simulink model "euler_equation_dave"  (R2021b)
settings: Solver=VariableStepAuto  StartTime=0.0  StopTime=30  MaxStep=0.01  RelTol=1e-3
values from neighbouring files (symbols this model uses):
  a = 2.4501e+4    (= 24501)    [heliocentric_plot.m]    (also in parameters_euler_equations_dave.m = 10500)
  e = 0.6665    [heliocentric_plot.m]    (also in parameters_euler_equations_dave.m = 0)
  Euler0131 = [0 pi/4 0]'    [parameters_euler_equations_dave.m]
  Euler0312 = [pi/4, 0, 0]'    [parameters_euler_equations_dave.m]
  h_versor = h ./ (h_norm)    [parameters_euler_equations_dave.m]
  I = [I_x_body, I_y_body, I_z_body]    [parameters_euler_equations_dave.m]
  i_0 = 0    [parameters_euler_equations_dave.m]
  J = diag (I)    [parameters_euler_equations_dave.m]
  J_inv = inv(J)    [parameters_euler_equations_dave.m]
  Mat_g = g .* S * 1e-09    [ghnorm.m]
  Mat_gsv = gsv .* S*  1e-09    [ghnorm.m]
  Mat_h = h .* S * 1e-09    [ghnorm.m]
  Mat_hsv = hsv .* S*  1e-09    [ghnorm.m]
  muP = astroConstants(13)    [parameters_euler_equations_dave.m]
  n = mat(:, 1)    [ghnorm.m]    (also in parameters_euler_equations_dave.m = 2*pi/T)
  N = max(mat (:, 2))    [ghnorm.m]    (also in parameters_euler_equations_dave.m = [n1 n2 n3 n4 n5 n6])
  n_sun = 2*pi/(365*24*3600)    (= 1.99238499086e-07)    [parameters_euler_equations_dave.m]    (also in srp.m = 1.99102127766e-07)
  R_sun = 149600000    [parameters_euler_equations_dave.m]
  Sat_dim = [a_body b_body c_body]    [parameters_euler_equations_dave.m]
  star1_in = [Sx(1); Sy(1); Sz(1)]    [parameters_euler_equations_dave.m]    (also in stars.m)
  star2_in = [Sx(2); Sy(2); Sz(2)]    [parameters_euler_equations_dave.m]    (also in stars.m)
  star3_in = [Sx(3); Sy(3); Sz(3)]    [parameters_euler_equations_dave.m]    (also in stars.m)
  theta_g0 = 0    [parameters_euler_equations_dave.m]
  true_anomaly0 = 0    [parameters_euler_equations_dave.m]
  Ts = 0.1    [parameters_euler_equations_dave.m]
  w0 = [wx, wy, wz]    [parameters_euler_equations_dave.m]
undefined symbols (not defined in the file or in its folder): A_SB, g_mat, h_mat, init_mjd2000, magnetic_torque, r0, t0, v0, vec_norm, we
libraries: sharedutil x13, vrlib x8, simulink_extras x6, sharedtransform x5, matrix_library x3, aerolibconvert2 x2, euler x1
(part 1 of 2)
settings Model: Creator=gargi  LastModifiedBy=white

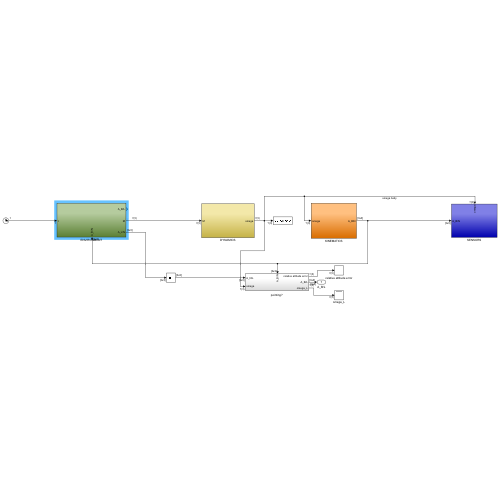
[thumbnail: Simulink's stored preview of the top-level diagram]
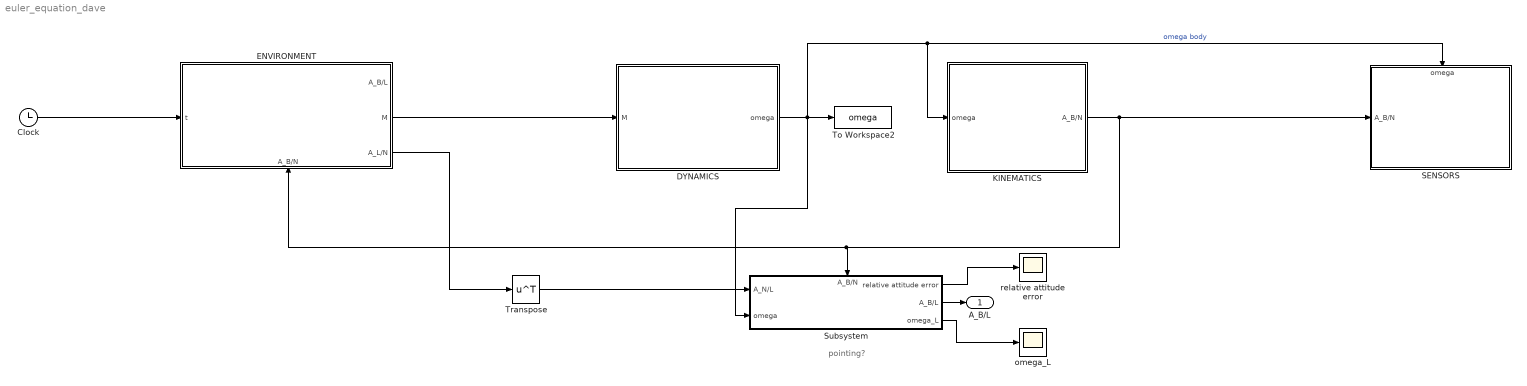
== system euler_equation_dave ==
  note: pointing?
  Clock : Clock
  DYNAMICS : Subsystem
  ENVIRONMENT : Subsystem
      settings: PortSchema="{\"entries\":[{\"content\":{\"sides\":[{\"content\":{\"connectorIds\":[\"In1\"]},\"type\":\"ConnectorPlacement.EquallySpacedRectSide\",\"uuid\":\"d64a220b-768f-41cc-b7f2-e1eda455b8cd\"},{\"content\":{\"connectorIds\":[\"Out1\",\"Out2\",\"Out3\"],\"side\":\"RIGHT\"},\"type\":\"ConnectorPlacement.EquallySpacedRectSide\",\"uuid\":\"0ef46d02-94aa-48e3-a1de-52aeb1814179\"},{\"content\":{\"connectorIds\":[],\"side\":\"TOP\"},\"type\":\"ConnectorPlacement.EquallySpacedRectSide\",\"uuid\":\"5be20339-a1cd-4229-b259-1b87d0a40b31\"},{\"content\":{\"connectorIds\":[\"In2\"],\"side\":\"BOTTOM\"},\"type\":\"ConnectorPlacement.EquallySpacedRectSide\",\"uuid\":\"00a59743-0b85-4da4-8c91-089e7d557d39\"}]},\"type\":\"ConnectorPlacement.EquallySpacedConnector\",\"uuid\":\"86e5647d-ad23-4d7e-bb48-80a2b4048e86\"}],\"packageUris\":[\"http://schema.mathworks.com/mf0/Connector/R2020b\"],\"version\":\"1.0\"}"
  KINEMATICS : Subsystem
  SENSORS : Subsystem
      settings: PortSchema="{\"entries\":[{\"content\":{\"sides\":[{\"content\":{\"connectorIds\":[\"In1\"]},\"type\":\"ConnectorPlacement.EquallySpacedRectSide\",\"uuid\":\"6630fbbb-ea2b-425d-8575-1523cccd696b\"},{\"content\":{\"connectorIds\":[],\"side\":\"RIGHT\"},\"type\":\"ConnectorPlacement.EquallySpacedRectSide\",\"uuid\":\"07965b78-7ff0-471d-b26c-4fdda1f5d939\"},{\"content\":{\"connectorIds\":[\"In2\"],\"side\":\"TOP\"},\"type\":\"ConnectorPlacement.EquallySpacedRectSide\",\"uuid\":\"40925145-5336-49f5-bea5-25b26df713fa\"}]},\"type\":\"ConnectorPlacement.EquallySpacedConnector\",\"uuid\":\"3c2f6bfd-4663-43ab-9562-77b2e75e3828\"}],\"packageUris\":[\"http://schema.mathworks.com/mf0/Connector/R2020b\"],\"version\":\"1.0\"}"
  Subsystem : Subsystem
      settings: PortSchema="{\"entries\":[{\"content\":{\"sides\":[{\"content\":{\"connectorIds\":[\"In1\",\"In2\"]},\"type\":\"ConnectorPlacement.EquallySpacedRectSide\",\"uuid\":\"153df774-f390-4caa-8633-d509b8614b34\"},{\"content\":{\"connectorIds\":[\"Out1\",\"Out2\",\"Out3\"],\"side\":\"RIGHT\"},\"type\":\"ConnectorPlacement.EquallySpacedRectSide\",\"uuid\":\"2b0b455d-aa9a-478c-9b12-a1c7f0c2757e\"},{\"content\":{\"connectorIds\":[\"In3\"],\"side\":\"TOP\"},\"type\":\"ConnectorPlacement.EquallySpacedRectSide\",\"uuid\":\"e181ccf7-3891-483c-b413-5a84ce39d941\"}]},\"type\":\"ConnectorPlacement.EquallySpacedConnector\",\"uuid\":\"4911c07f-3db9-4f8f-9913-f96600dbf3f5\"}],\"packageUris\":[\"http://schema.mathworks.com/mf0/Connector/R2020b\"],\"version\":\"1.0\"}"
  To Workspace2 : ToWorkspace  VariableName=omega  SampleTime=-1
  Transpose : Math  Operator=transpose  SaturateOnIntegerOverflow=on
  omega_L : Scope
  relative attitude error : Scope
  A_B/L : Outport
  wires:
  DYNAMICS/1(omega) -> To Workspace2/1, SENSORS/2(omega), KINEMATICS/1(omega), Subsystem/2(omega)  "omega body"
  KINEMATICS/1(A_B/N) -> SENSORS/1(A_B/N), Subsystem/3(A_B/N), ENVIRONMENT/2(A_B/N)
  Transpose/1 -> Subsystem/1(A_N/L)
  Subsystem/1(relative attitude error) -> relative attitude error/1
  Subsystem/2(A_B/L) -> A_B/L/1
  Subsystem/3(omega_L) -> omega_L/1
  ENVIRONMENT/3(A_L/N) -> Transpose/1
  ENVIRONMENT/2(M) -> DYNAMICS/1(M)
  Clock/1 -> ENVIRONMENT/1(t)

== system euler_equation_dave/DYNAMICS ==
  M : Inport
  Cross Product : matrix_library/Cross Product
      settings: SourceProductBaseCode=SL
  Integrator : Integrator  InitialCondition=w0
  J : Gain  Gain=J  Multiplication=Matrix(K*u)
  J inv : Gain  Gain=J_inv  Multiplication=Matrix(K*u)
  Sum : Sum  Inputs=|++
  omega : Outport
  wires:
  Integrator/1 -> J/1, Cross Product/2, omega/1
  J/1 -> Cross Product/1
  J inv/1 -> Integrator/1  "omega_dot"
  Cross Product/1 -> Sum/1  "J w cross w"
  Sum/1 -> J inv/1
  M/1 -> Sum/2

== system euler_equation_dave/ENVIRONMENT ==
  note: A is from INERTIAL to LVLH
  t : Inport
  A_B/N : Inport  Port=2
  ECEF : Subsystem
  GRADIENT TORQUE : Subsystem
  MAGNETIC TORQUE : Subsystem
  "ORBITAL MECHANICS " : Subsystem
  SRP : Subsystem  Commented=on
  SUN : Subsystem
  Scope : Scope
  Scope1 : Scope
  Sum : Sum  Inputs=+++
  To create A_L/N : Subsystem
  h : Constant  Value=h_versor
  "to create c1, c2, c3" : Subsystem
  A_B/L : Outport
  M : Outport  Port=2
  A_L/N : Outport  Port=3
  wires:
  "to create c1, c2, c3"/1("c1, c2, c3") -> GRADIENT TORQUE/1("c1, c2, c3")  "c1,c2,c3"
  A_B/N/1 -> SRP/1(A_BN), SUN/1(A_BN), MAGNETIC TORQUE/2(A_B/N), "to create c1, c2, c3"/1(A_B/N)
  "to create c1, c2, c3"/2(A_B/L) -> A_B/L/1
  GRADIENT TORQUE/1(M_GG) -> Sum/1
  Sum/1 -> M/1
  To create A_L/N/1(A_L/N) -> Scope/1, A_L/N/1, "to create c1, c2, c3"/2(A_L/N)
  h/1 -> To create A_L/N/1(h_versor)
  "ORBITAL MECHANICS "/2(R) -> GRADIENT TORQUE/2(R)  "in km"
  "ORBITAL MECHANICS "/1(r_N_versor) -> To create A_L/N/2(r_N_versor)
  t/1 -> SUN/2(t), MAGNETIC TORQUE/3(t), SRP/2(t)
  SRP/1(Output) -> Scope1/1, Sum/3
  "ORBITAL MECHANICS "/4(r_N) -> MAGNETIC TORQUE/1(r_N)  "r_N in km"
  MAGNETIC TORQUE/1(M_Magn) -> Sum/2

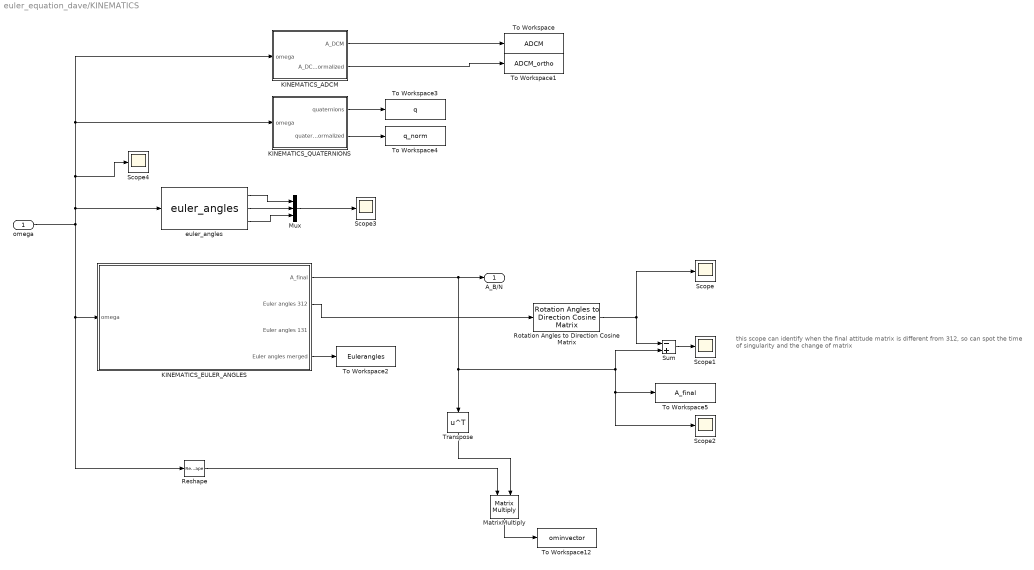
== system euler_equation_dave/KINEMATICS ==
  note: this scope can identify when the final attitude
      | matrix is different from 312, so can spot
      | the time of singularity and the change of matrix
  omega : Inport
  KINEMATICS_ADCM : Subsystem
  KINEMATICS_EULER_ANGLES : Subsystem
  KINEMATICS_QUATERNIONS : Subsystem
  MatrixMultiply : Product  Multiplication=Matrix(*)
  Mux : Mux  Inputs=3
  Reshape : Reshape  OutputDimensionality=Row vector (2-D)
  Rotation Angles to Direction Cosine Matrix : sharedtransform/Rotation Angles to Direction Cosine Matrix  rotationOrder=ZXY  aMode=aMode
      settings: SourceProductBaseCode=AE,PW,DR,MT,UV,VE
  Scope{,1..4} (5 alike) : Scope
  Sum : Sum  Inputs=-+
  To Workspace : ToWorkspace  VariableName=ADCM  SampleTime=-1
  To Workspace1 : ToWorkspace  VariableName=ADCM_ortho  SampleTime=-1
  To Workspace12 : ToWorkspace  VariableName=ominvector  SampleTime=-1
  To Workspace2 : ToWorkspace  VariableName=Eulerangles  SampleTime=-1
  To Workspace3 : ToWorkspace  VariableName=q  SampleTime=-1
  To Workspace4 : ToWorkspace  VariableName=q_norm  SampleTime=-1
  To Workspace5 : ToWorkspace  VariableName=A_final  SampleTime=-1
  Transpose : Math  Operator=transpose  SaturateOnIntegerOverflow=on
  euler_angles : euler/euler_angles  SystemSampleTime=-1  VariantActivationTime=update diagram  Latency=0  AutoFrameSizeCalculation=off
      link override phi_block/Integrator: InitialCondition=pi/4
      link override psi_block/Integrator: InitialCondition=0
      link override theta_block/Integrator: InitialCondition=0
  A_B/N : Outport
  wires:
  Transpose/1 -> MatrixMultiply/2
  Reshape/1 -> MatrixMultiply/1
  KINEMATICS_QUATERNIONS/2(quaternions normalized) -> To Workspace4/1
  omega/1 -> euler_angles/1, Scope4/1, KINEMATICS_ADCM/1(omega), KINEMATICS_QUATERNIONS/1(omega), KINEMATICS_EULER_ANGLES/1(omega), Reshape/1
  MatrixMultiply/1 -> To Workspace12/1
  KINEMATICS_ADCM/2(A_DCM orthonormalized) -> To Workspace1/1
  KINEMATICS_QUATERNIONS/1(quaternions) -> To Workspace3/1
  KINEMATICS_EULER_ANGLES/1(A_final) -> Scope2/1, To Workspace5/1, Sum/2, Transpose/1, A_B/N/1
  KINEMATICS_ADCM/1(A_DCM) -> To Workspace/1
  Sum/1 -> Scope1/1
  KINEMATICS_EULER_ANGLES/2(Euler angles 312) -> Rotation Angles to Direction Cosine Matrix/1
  Rotation Angles to Direction Cosine Matrix/1 -> Scope/1, Sum/1
  KINEMATICS_EULER_ANGLES/4(Euler angles merged) -> To Workspace2/1
  euler_angles/1 -> Mux/1
  euler_angles/2 -> Mux/2
  euler_angles/3 -> Mux/3
  Mux/1 -> Scope3/1

== system euler_equation_dave/SENSORS ==
  A_B/N : Inport
  omega : Inport  Port=2
  ATTITUDE DETERMINATION FOR GYROSCOPES : Subsystem  Commented=on
  ATTITUDE DETERMINATION FOR STAR SENSOR : Subsystem  Commented=on
  GYROSCOPES : Subsystem  Commented=on
  STAR SENSOR : Subsystem  Commented=on
  wires:
  omega/1 -> GYROSCOPES/1(omega)
  A_B/N/1 -> STAR SENSOR/1(A_B/N)
  GYROSCOPES/1(omega measured) -> ATTITUDE DETERMINATION FOR GYROSCOPES/1(omega measured)
  ATTITUDE DETERMINATION FOR GYROSCOPES/1(Attitude final measured) -> ?
  ATTITUDE DETERMINATION FOR GYROSCOPES/2(Euler angles merged measured) -> ?
  STAR SENSOR/1(star1_meas) -> ?
  STAR SENSOR/2(star2_meas) -> ?

== system euler_equation_dave/Subsystem ==
  A_N/L : Inport
  omega : Inport  Port=2
  A_B/N : Inport  Port=3
  MatrixMultiply : Product  Multiplication=Matrix(*)
  MatrixMultiply1 : Product  Multiplication=Matrix(*)
  MatrixMultiply2 : Product  Multiplication=Matrix(*)
  Scope : Scope
  Sum : Sum  Inputs=+-
  Transpose1 : Math  Operator=transpose  SaturateOnIntegerOverflow=on
  relative attitude error : Outport
  A_B/L : Outport  Port=2
  omega_L : Outport  Port=3
  wires:
  MatrixMultiply/1 -> Transpose1/1, MatrixMultiply2/1, A_B/L/1  "A_B/L"
  Transpose1/1 -> MatrixMultiply1/1  "A_L/B"
  omega/1 -> Sum/1, MatrixMultiply1/2  "omega"
  MatrixMultiply1/1 -> omega_L/1, MatrixMultiply2/2, Sum/2  "omega_L"
  A_B/N/1 -> MatrixMultiply/1
  A_N/L/1 -> MatrixMultiply/2
  Sum/1 -> relative attitude error/1

== system euler_equation_dave/ENVIRONMENT/ECEF ==
  In1 : Inport
  Out1 : Outport
  wires:
  In1/1 -> Out1/1

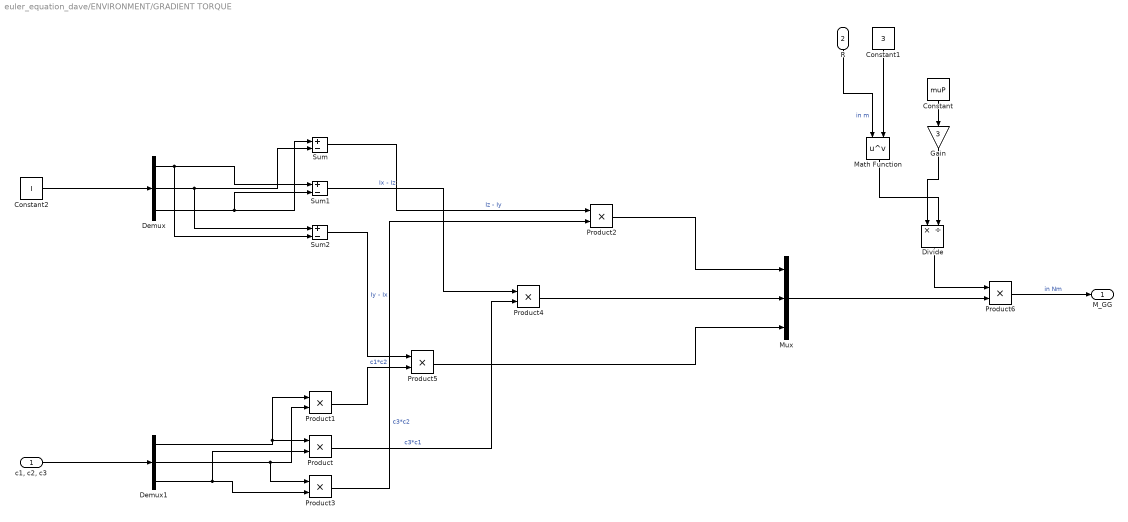
== system euler_equation_dave/ENVIRONMENT/GRADIENT TORQUE ==
  "c1, c2, c3" : Inport
  R : Inport  Port=2
  Constant : Constant  Value=muP
  Constant1 : Constant  Value=3
  Constant2 : Constant  Value=I
  Demux : Demux  Outputs=3
  Demux1 : Demux  Outputs=3
  Divide : Product  Inputs=*/
  Gain : Gain  Gain=3
  Math Function : Math  Operator=pow  SaturateOnIntegerOverflow=on
  Mux : Mux  Inputs=3
  Product{,1..6} (7 alike) : Product
  Sum : Sum  Inputs=+-
  Sum1 : Sum  Inputs=+-
  Sum2 : Sum  Inputs=+-
  M_GG : Outport
  wires:
  Constant/1 -> Gain/1
  Gain/1 -> Divide/1
  R/1 -> Math Function/1  "in m"
  Constant1/1 -> Math Function/2
  Math Function/1 -> Divide/2
  Constant2/1 -> Demux/1
  Demux/1 -> Sum2/2, Sum1/1
  Demux/2 -> Sum2/1, Sum/2
  Demux/3 -> Sum/1, Sum1/2
  Demux1/1 -> Product1/1, Product/1
  Demux1/2 -> Product1/2, Product3/1
  Demux1/3 -> Product/2, Product3/2
  "c1, c2, c3"/1 -> Demux1/1
  Sum/1 -> Product2/1  "Iz - Iy"
  Sum1/1 -> Product4/1  "Ix - Iz"
  Product3/1 -> Product2/2  "c3*c2"
  Product/1 -> Product4/2  "c3*c1"
  Product1/1 -> Product5/2  "c1*c2"
  Sum2/1 -> Product5/1  "Iy - Ix"
  Product2/1 -> Mux/1
  Product5/1 -> Mux/3
  Product4/1 -> Mux/2
  Divide/1 -> Product6/1
  Mux/1 -> Product6/2
  Product6/1 -> M_GG/1  "in Nm"

== system euler_equation_dave/ENVIRONMENT/MAGNETIC TORQUE ==
  r_N : Inport
  A_B/N : Inport  Port=2
  t : Inport  Port=3
  Subsystem : Subsystem  Commented=on
  magnetic_torque : Subsystem  AncestorBlock=magnetic_torque/magnetic_torque
  M_Magn : Outport
  wires:
  r_N/1 -> magnetic_torque/1(r_N)
  A_B/N/1 -> magnetic_torque/2(A_N_to_B)
  magnetic_torque/1(magnetic_torque) -> M_Magn/1
  t/1 -> magnetic_torque/3(t)

== system euler_equation_dave/ENVIRONMENT/ORBITAL MECHANICS  ==
  Scope1 : Scope
  Sum : Sum  Inputs=+-
  cartesian position integrator : Subsystem
  "cartesian position with keplerian formulas " : Subsystem
  r_N_versor : Outport
  R : Outport  Port=2
  cartesian position : Outport  Port=3
  r_N : Outport  Port=4
  wires:
  Sum/1 -> Scope1/1
  cartesian position integrator/1(carteasion_position_versor) -> Sum/2
  cartesian position integrator/2(cartesian position) -> cartesian position/1
  "cartesian position with keplerian formulas "/3(r_N_versor) -> Sum/1, r_N_versor/1
  "cartesian position with keplerian formulas "/1(R) -> R/1
  "cartesian position with keplerian formulas "/2(rN) -> r_N/1

== system euler_equation_dave/ENVIRONMENT/SRP ==
  A_BN : Inport
  t : Inport  Port=2
  MATLAB Function : MATLAB Function  TreatAsAtomicUnit=on
  N_surfaces : Constant  Value=N
  Reshape : Reshape
  Sat_dim : Constant  Value=Sat_dim
  Output : Outport
  wires:
  Sat_dim/1 -> MATLAB Function/1(Sat_dim)
  t/1 -> MATLAB Function/4(t)  "clock"
  A_BN/1 -> MATLAB Function/3(A_BN)
  N_surfaces/1 -> MATLAB Function/2(N)
  MATLAB Function/1(M) -> Reshape/1
  Reshape/1 -> Output/1

== system euler_equation_dave/ENVIRONMENT/SUN ==
  A_BN : Inport
  t : Inport  Port=2
  Constant2 : Constant  Value=eps
  Cos : Trigonometry  Operator=cos
  Cos1 : Trigonometry  Operator=cos
  Gain : Gain  Gain=R_sun
  MatrixMultiply : Product  Multiplication=Matrix(*)
  Mux : Mux  Inputs=3
  Normalize Vector : vrlib/Utilities/Normalize Vector  maxzero=0
  Product1 : Product
  Product2 : Product
  Sin : Trigonometry
  Sin1 : Trigonometry
  "n_sun " : Gain  Gain=n_sun
  S_N : Outport  VectorParamsAs1DForOutWhenUnconnected=off
  S_B : Outport  Port=2
  wires:
  Mux/1 -> Gain/1
  Product2/1 -> Mux/3
  Product1/1 -> Mux/2
  Cos/1 -> Mux/1
  t/1 -> "n_sun "/1
  Constant2/1 -> Sin1/1, Cos1/1
  Sin1/1 -> Product2/2
  Sin/1 -> Product1/1, Product2/1
  "n_sun "/1 -> Sin/1, Cos/1
  Cos1/1 -> Product1/2
  Gain/1 -> Normalize Vector/1
  A_BN/1 -> MatrixMultiply/1
  Normalize Vector/1 -> MatrixMultiply/2, S_N/1
  MatrixMultiply/1 -> S_B/1

== system euler_equation_dave/ENVIRONMENT/To create A_L//N ==
  h_versor : Inport
  r_N_versor : Inport  Port=2
  Create 3x3 Matrix : sharedutil/Create 3x3 Matrix  aMode=aMode
      settings: SourceProductBaseCode=AE,PW,DR,MT,UV,VE
  Demux : Demux  Outputs=3
  Demux1 : Demux  Outputs=3
  Demux2 : Demux  Outputs=3
  Scope : Scope
  To comput theta_versor : Subsystem
  A_L/N : Outport
  wires:
  Demux2/3 -> Create 3x3 Matrix/9
  Demux/1 -> Create 3x3 Matrix/1
  r_N_versor/1 -> To comput theta_versor/2(r_N_versor), Demux/1
  Demux/3 -> Create 3x3 Matrix/3
  To comput theta_versor/1(theta_versor) -> Demux1/1
  Demux2/2 -> Create 3x3 Matrix/8
  Demux1/1 -> Create 3x3 Matrix/4
  Demux2/1 -> Create 3x3 Matrix/7
  Demux/2 -> Create 3x3 Matrix/2
  Demux1/2 -> Create 3x3 Matrix/5
  Demux1/3 -> Create 3x3 Matrix/6
  h_versor/1 -> Demux2/1, To comput theta_versor/1(h_versor)
  Create 3x3 Matrix/1 -> Scope/1, A_L/N/1

== system euler_equation_dave/ENVIRONMENT/to create c1, c2, c3 ==
  note: from LVLH to Body frame
  A_B/N : Inport
  A_L/N : Inport  Port=2
  Constant : Constant  Value=[1 0 0]'
  MatrixMultiply : Product  Multiplication=Matrix(*)
  MatrixMultiply1 : Product  Multiplication=Matrix(*)
  Transpose : Math  Operator=transpose  SaturateOnIntegerOverflow=on
  "c1, c2, c3" : Outport
  A_B/L : Outport  Port=2
  wires:
  MatrixMultiply/1 -> A_B/L/1, MatrixMultiply1/1
  A_L/N/1 -> Transpose/1
  Constant/1 -> MatrixMultiply1/2
  Transpose/1 -> MatrixMultiply/2
  MatrixMultiply1/1 -> "c1, c2, c3"/1  "c1, c2, c3"
  A_B/N/1 -> MatrixMultiply/1

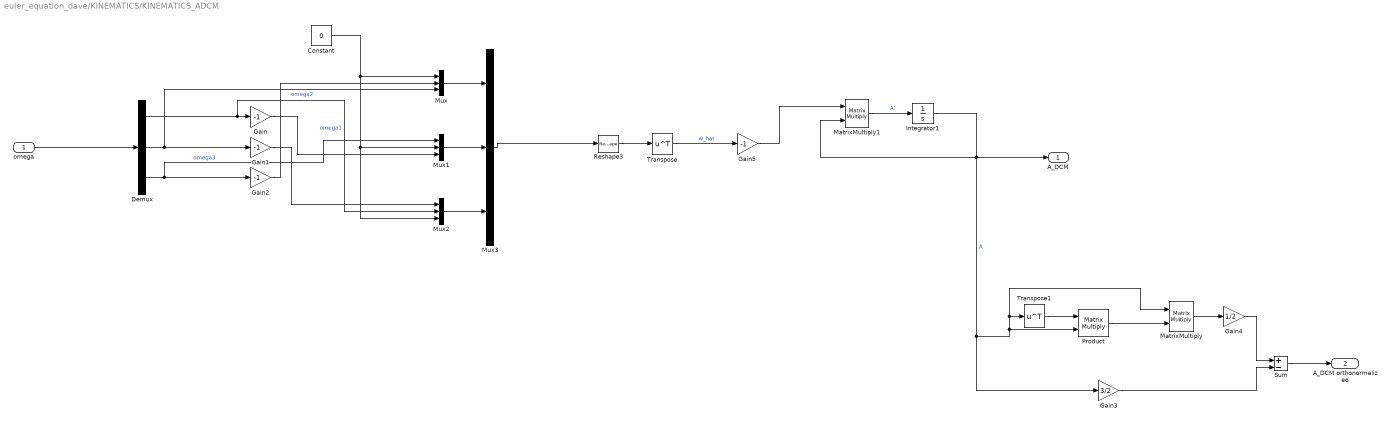
== system euler_equation_dave/KINEMATICS/KINEMATICS_ADCM ==
  omega : Inport
  Constant : Constant  Value=0
  Demux : Demux  Outputs=3
  Gain{,1..2,5} (4 alike) : Gain  Gain=-1
  Gain3 : Gain  Gain=3/2
  Gain4 : Gain  Gain=1/2
  Integrator1 : Integrator  InitialCondition=eye(3)
  MatrixMultiply : Product  Multiplication=Matrix(*)
  MatrixMultiply1 : Product  Multiplication=Matrix(*)
  Mux{,1..3} (4 alike) : Mux  Inputs=3
  Product : Product  Multiplication=Matrix(*)
  Reshape3 : Reshape  OutputDimensionality=Customize  OutputDimensions=[3 3]
  Sum : Sum  Inputs=+-
  Transpose : Math  Operator=transpose  SaturateOnIntegerOverflow=on
  Transpose1 : Math  Operator=transpose  SaturateOnIntegerOverflow=on
  A_DCM : Outport
  A_DCM orthonormalized : Outport  Port=2
  wires:
  Mux/1 -> Mux3/1
  Demux/1 -> Gain/1, Mux2/2  "omega1"
  Constant/1 -> Mux2/3, Mux1/2, Mux/1
  Gain/1 -> Mux1/3
  Mux3/1 -> Reshape3/1
  Gain1/1 -> Mux2/1
  Demux/2 -> Mux/3, Gain1/1  "omega2"
  Mux1/1 -> Mux3/2
  Demux/3 -> Mux1/1, Gain2/1  "omega3"
  Mux2/1 -> Mux3/3
  Gain2/1 -> Mux/2
  Reshape3/1 -> Transpose/1
  omega/1 -> Demux/1
  Transpose/1 -> Gain5/1  "w_hat"
  Integrator1/1 -> MatrixMultiply1/2, A_DCM/1, MatrixMultiply/1, Transpose1/1, Product/2, Gain3/1  "A"
  Transpose1/1 -> Product/1
  Gain4/1 -> Sum/1
  Gain3/1 -> Sum/2
  Sum/1 -> A_DCM orthonormalized/1
  MatrixMultiply/1 -> Gain4/1
  Product/1 -> MatrixMultiply/2
  Gain5/1 -> MatrixMultiply1/1
  MatrixMultiply1/1 -> Integrator1/1  "A'"

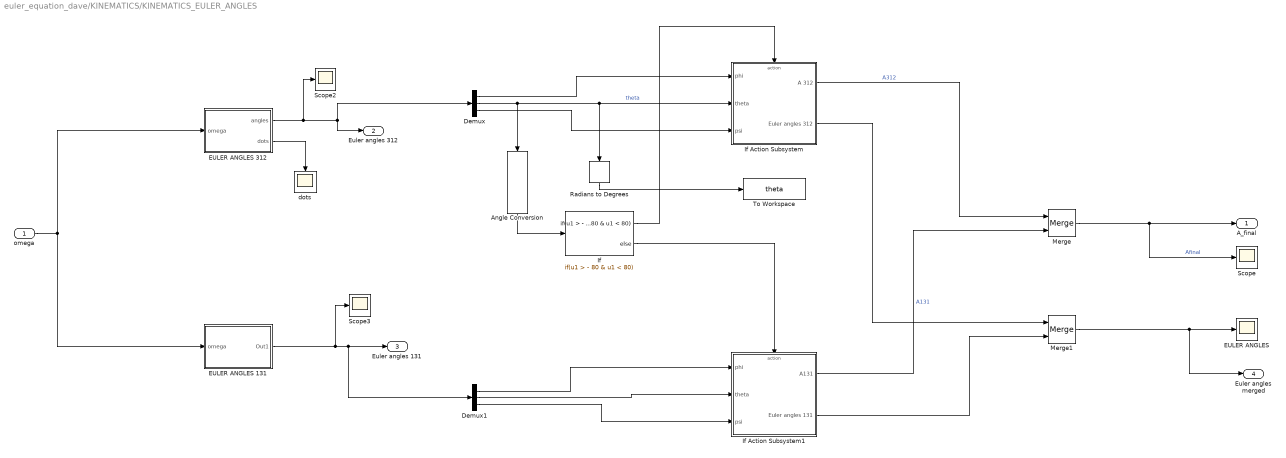
== system euler_equation_dave/KINEMATICS/KINEMATICS_EULER_ANGLES ==
  omega : Inport
  Angle Conversion : aerolibconvert2/Angle Conversion  IU=rad  OU=deg
  Demux : Demux  Outputs=3
  Demux1 : Demux  Outputs=3
  EULER ANGLES : Scope
  EULER ANGLES 131 : Subsystem
  EULER ANGLES 312 : Subsystem
  If : If  IfExpression=u1 > - 80 & u1 < 80
  If Action Subsystem : Subsystem  TreatAsAtomicUnit=on
  If Action Subsystem1 : Subsystem  TreatAsAtomicUnit=on
  Merge : Merge
  Merge1 : Merge
  Radians to Degrees : simulink_extras/Transformations/Radians to Degrees
  Scope : Scope
  Scope2 : Scope
  Scope3 : Scope
  To Workspace : ToWorkspace  VariableName=theta  SaveFormat=Timeseries  SampleTime=-1
  dots : Scope
  A_final : Outport
  Euler angles 312 : Outport  Port=2
  Euler angles 131 : Outport  Port=3
  Euler angles merged : Outport  Port=4
  wires:
  Angle Conversion/1 -> If/1
  If/2 -> If Action Subsystem1/Action
  If/1 -> If Action Subsystem/Action
  If Action Subsystem1/1(A131) -> Merge/2  "A131"
  If Action Subsystem/1(A 312) -> Merge/1  "A312"
  Merge/1 -> Scope/1, A_final/1  "Afinal"
  omega/1 -> EULER ANGLES 312/1(omega), EULER ANGLES 131/1(omega)
  Demux/2 -> Radians to Degrees/1, If Action Subsystem/2(theta), Angle Conversion/1  "theta"
  Demux/1 -> If Action Subsystem/1(phi)
  Demux/3 -> If Action Subsystem/3(psi)
  EULER ANGLES 312/1(angles) -> Scope2/1, Euler angles 312/1, Demux/1
  Demux1/1 -> If Action Subsystem1/1(phi)
  Demux1/2 -> If Action Subsystem1/2(theta)
  Demux1/3 -> If Action Subsystem1/3(psi)
  EULER ANGLES 131/1(Out1) -> Scope3/1, Euler angles 131/1, Demux1/1
  If Action Subsystem/2(Euler angles 312) -> Merge1/1
  If Action Subsystem1/2(Euler angles 131) -> Merge1/2
  Merge1/1 -> Euler angles merged/1, EULER ANGLES/1
  EULER ANGLES 312/2(dots) -> dots/1
  Radians to Degrees/1 -> To Workspace/1

== system euler_equation_dave/KINEMATICS/KINEMATICS_QUATERNIONS ==
  omega : Inport
  Demux : Demux  Outputs=3
  Gain : Gain  Gain=1/2
  Integrator : Integrator  InitialCondition=[0 0 0 1]
  Normalize Vector : vrlib/Utilities/Normalize Vector  maxzero=0
  Product : Product
  Product1 : Product
  Product2 : Product
  Product3 : Product  Multiplication=Matrix(*)
  Sum : Sum  Inputs=+++
  mat1 : Constant  Value=[0 0 0 1; 0 0 1 0; 0 -1 0 0; -1 0 0 0]
  mat2 : Constant  Value=[0 0 -1 0; 0 0 0 1; 1 0 0 0; 0 -1 0 0]
  mat3 : Constant  Value=[0 1 0 0; -1 0 0 0; 0 0 0 1; 0 0 -1 0]
  quaternions : Outport
  quaternions normalized : Outport  Port=2
  wires:
  mat1/1 -> Product/1
  Demux/1 -> Product/2
  Product/1 -> Sum/1
  mat2/1 -> Product1/1
  Demux/2 -> Product1/2
  Product1/1 -> Sum/2
  Demux/3 -> Product2/2
  mat3/1 -> Product2/1
  Product2/1 -> Sum/3
  Sum/1 -> Gain/1  "OMEGA"
  omega/1 -> Demux/1
  Gain/1 -> Product3/1
  Product3/1 -> Integrator/1  "q'"
  Integrator/1 -> quaternions/1, Normalize Vector/1  "q"
  Normalize Vector/1 -> Product3/2, quaternions normalized/1

== system euler_equation_dave/SENSORS/ATTITUDE DETERMINATION FOR GYROSCOPES ==
  note: star sensor
  omega measured : Inport
  Angle Conversion : aerolibconvert2/Angle Conversion  IU=rad  OU=deg
  Demux : Demux  Outputs=3
  Demux1 : Demux  Outputs=3
  EULER ANGLES : Scope
  EULER ANGLES 131 : Subsystem
  EULER ANGLES 312 : Subsystem
  If : If  IfExpression=u1 > - 80 & u1 < 80
  If Action Subsystem : Subsystem  TreatAsAtomicUnit=on
  If Action Subsystem1 : Subsystem  TreatAsAtomicUnit=on
  Merge : Merge
  Merge1 : Merge
  Scope : Scope
  Scope2 : Scope
  Scope3 : Scope
  dots : Scope
  Attitude final measured : Outport
  Euler angles merged measured : Outport  Port=2
  wires:
  If Action Subsystem1/1(A131) -> Merge/2  "A131"
  EULER ANGLES 312/2(dots) -> dots/1
  EULER ANGLES 131/1(Out1) -> Scope3/1, Demux1/1
  Demux1/2 -> If Action Subsystem1/2(theta)
  Demux1/3 -> If Action Subsystem1/3(psi)
  Demux/1 -> If Action Subsystem/1(phi)
  Demux/3 -> If Action Subsystem/3(psi)
  Merge/1 -> Scope/1, Attitude final measured/1  "Afinal"
  If Action Subsystem1/2(Euler angles 131) -> Merge1/2
  Demux1/1 -> If Action Subsystem1/1(phi)
  omega measured/1 -> EULER ANGLES 312/1(omega), EULER ANGLES 131/1(omega)
  Merge1/1 -> Euler angles merged measured/1, EULER ANGLES/1
  If Action Subsystem/2(Euler angles 312) -> Merge1/1
  Demux/2 -> If Action Subsystem/2(theta), Angle Conversion/1  "theta"
  If Action Subsystem/1(A 312) -> Merge/1  "A312"
  EULER ANGLES 312/1(angles) -> Scope2/1, Demux/1
  Angle Conversion/1 -> If/1
  If/1 -> If Action Subsystem/Action
  If/2 -> If Action Subsystem1/Action

== system euler_equation_dave/SENSORS/ATTITUDE DETERMINATION FOR STAR SENSOR ==
  In1 : Inport
  Out1 : Outport
  wires:
  In1/1 -> Out1/1

== system euler_equation_dave/SENSORS/GYROSCOPES ==
  omega : Inport
  Bias : Constant  Value=[1; 1; 1]*0.0035
  Degrees to Radians : simulink_extras/Transformations/Degrees to Radians
  Gain : Gain  Gain=1/3600
  Product : Product
  Random Number : RandomNumber  Mean=[0 0 0 ]'  Variance=[1 1 1]'  Seed=[0 0 0]'  SampleTime=0.1
  Scope1 : Scope
  Scope2 : Scope
  Sigma_n : Subsystem
  Sum : Sum  Inputs=+++
  Sum1 : Sum  Inputs=+-
  omega measured : Outport
  wires:
  Bias/1 -> Degrees to Radians/1  "b in deg/h"
  Degrees to Radians/1 -> Gain/1
  Sum/1 -> omega measured/1, Sum1/1
  omega/1 -> Scope2/1, Sum1/2, Sum/2
  Gain/1 -> Sum/3
  Sum1/1 -> Scope1/1
  Random Number/1 -> Product/2
  Product/1 -> Sum/1
  Sigma_n/1(Out1) -> Product/1

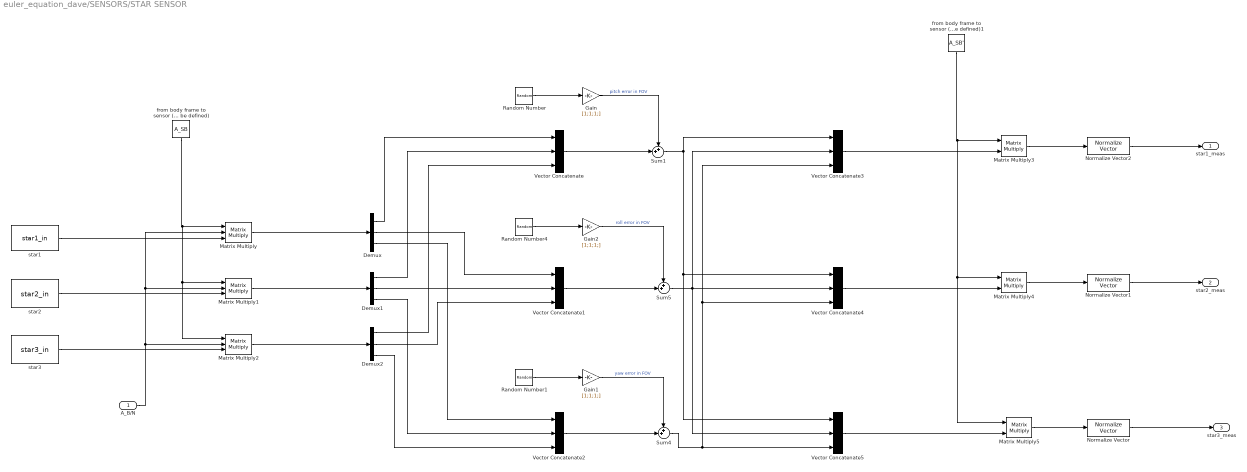
== system euler_equation_dave/SENSORS/STAR SENSOR ==
  A_B/N : Inport
  Demux : Demux  Outputs=3
  Demux1 : Demux  Outputs=3
  Demux2 : Demux  Outputs=3
  Gain : Gain  Gain=[1;1;1;]
  Gain1 : Gain  Gain=[1;1;1;]
  Gain2 : Gain  Gain=[1;1;1;]
  Matrix Multiply : Product  Inputs=3  Multiplication=Matrix(*)
  Matrix Multiply1 : Product  Inputs=3  Multiplication=Matrix(*)
  Matrix Multiply2 : Product  Inputs=3  Multiplication=Matrix(*)
  Matrix Multiply3 : Product  Multiplication=Matrix(*)
  Matrix Multiply4 : Product  Multiplication=Matrix(*)
  Matrix Multiply5 : Product  Multiplication=Matrix(*)
  Normalize Vector : vrlib/Utilities/Normalize Vector  maxzero=0
  Normalize Vector1 : vrlib/Utilities/Normalize Vector  maxzero=0
  Normalize Vector2 : vrlib/Utilities/Normalize Vector  maxzero=0
  Random Number : RandomNumber  Variance=((8.25/3600)*(pi/180))^2  SampleTime=0.1
  Random Number1 : RandomNumber  Variance=((8.25/3600)*(pi/180))^2  SampleTime=0.1
  Random Number4 : RandomNumber  Variance=((11.1/3600)*(pi/180))^2  SampleTime=0.1
  Sum1 : Sum  Inputs=++|
  Sum4 : Sum  Inputs=++|
  Sum5 : Sum  Inputs=++|
  Vector Concatenate{,1..5} (6 alike) : Concatenate  NumInputs=3
  from body frame to sensor (yet to be defined) : Constant  Value=A_SB
  from body frame to sensor (yet to be defined)1 : Constant  Value=A_SB'
  star1 : Constant  Value=star1_in
  star2 : Constant  Value=star2_in
  star3 : Constant  Value=star3_in
  star1_meas : Outport
  star2_meas : Outport  Port=2
  star3_meas : Outport  Port=3
  wires:
  Demux/1 -> Vector Concatenate/1
  Demux1/1 -> Vector Concatenate/2
  Demux2/1 -> Vector Concatenate/3
  Demux/2 -> Vector Concatenate1/1
  Demux1/2 -> Vector Concatenate1/2
  Demux2/2 -> Vector Concatenate1/3
  Demux/3 -> Vector Concatenate2/1
  Demux1/3 -> Vector Concatenate2/2
  Demux2/3 -> Vector Concatenate2/3
  Matrix Multiply/1 -> Demux/1
  Matrix Multiply1/1 -> Demux1/1
  Matrix Multiply2/1 -> Demux2/1
  A_B/N/1 -> Matrix Multiply/2, Matrix Multiply1/2, Matrix Multiply2/2
  from body frame to sensor (yet to be defined)/1 -> Matrix Multiply2/1, Matrix Multiply1/1, Matrix Multiply/1
  star1/1 -> Matrix Multiply/3
  star2/1 -> Matrix Multiply1/3
  star3/1 -> Matrix Multiply2/3
  Vector Concatenate/1 -> Sum1/2
  Random Number/1 -> Gain/1
  Gain/1 -> Sum1/1  "pitch error in FOV"
  Random Number4/1 -> Gain2/1
  Gain2/1 -> Sum5/1  "roll error in FOV"
  Vector Concatenate1/1 -> Sum5/2
  Random Number1/1 -> Gain1/1
  Gain1/1 -> Sum4/1  "yaw error in FOV"
  Vector Concatenate2/1 -> Sum4/2
  Sum1/1 -> Vector Concatenate3/1, Vector Concatenate5/1, Vector Concatenate4/1
  Sum5/1 -> Vector Concatenate5/2, Vector Concatenate4/2, Vector Concatenate3/2
  Sum4/1 -> Vector Concatenate4/3, Vector Concatenate3/3, Vector Concatenate5/3
  Vector Concatenate3/1 -> Matrix Multiply3/2
  Vector Concatenate4/1 -> Matrix Multiply4/2
  Vector Concatenate5/1 -> Matrix Multiply5/2
  from body frame to sensor (yet to be defined)1/1 -> Matrix Multiply3/1, Matrix Multiply4/1, Matrix Multiply5/1
  Matrix Multiply3/1 -> Normalize Vector2/1
  Normalize Vector2/1 -> star1_meas/1
  Matrix Multiply4/1 -> Normalize Vector1/1
  Normalize Vector1/1 -> star2_meas/1
  Matrix Multiply5/1 -> Normalize Vector/1
  Normalize Vector/1 -> star3_meas/1

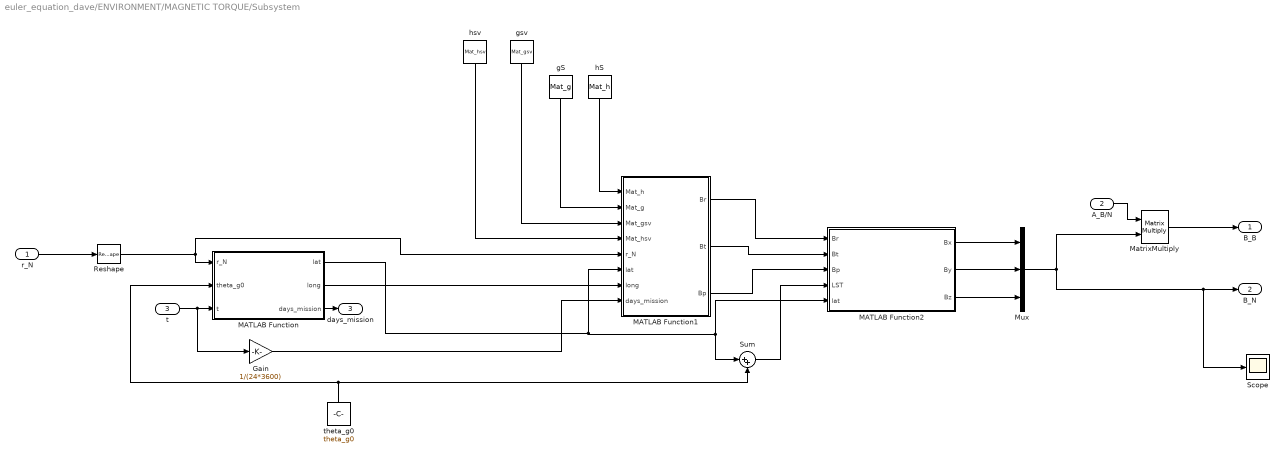
== system euler_equation_dave/ENVIRONMENT/MAGNETIC TORQUE/Subsystem ==
  r_N : Inport
  A_B/N : Inport  Port=2
  t : Inport  Port=3
  Gain : Gain  Gain=1/(24*3600)
  MATLAB Function : MATLAB Function  TreatAsAtomicUnit=on
  MATLAB Function1 : MATLAB Function  TreatAsAtomicUnit=on
  MATLAB Function2 : MATLAB Function  TreatAsAtomicUnit=on
  MatrixMultiply : Product  Multiplication=Matrix(*)
  Mux : Mux  Inputs=3
  Reshape : Reshape  OutputDimensionality=Row vector (2-D)
  Scope : Scope
  Sum : Sum  Inputs=|++
  gS : Constant  Value=Mat_g
  gsv : Constant  Value=Mat_gsv
  hS : Constant  Value=Mat_h
  hsv : Constant  Value=Mat_hsv
  theta_g0 : Constant  Value=theta_g0
  B_B : Outport
  B_N : Outport  Port=2
  days_mission : Outport  Port=3
  wires:
  MATLAB Function/2(long) -> MATLAB Function1/7(long)
  A_B/N/1 -> MatrixMultiply/1
  MATLAB Function2/1(Bx) -> Mux/1
  MATLAB Function2/2(By) -> Mux/2
  MATLAB Function2/3(Bz) -> Mux/3
  MATLAB Function1/1(Br) -> MATLAB Function2/1(Br)
  theta_g0/1 -> MATLAB Function/2(theta_g0), Sum/2
  MATLAB Function1/2(Bt) -> MATLAB Function2/2(Bt)
  MATLAB Function1/3(Bp) -> MATLAB Function2/3(Bp)
  MATLAB Function/1(lat) -> MATLAB Function1/6(lat), Sum/1, MATLAB Function2/5(lat)
  Sum/1 -> MATLAB Function2/4(LST)
  MatrixMultiply/1 -> B_B/1
  gsv/1 -> MATLAB Function1/3(Mat_gsv)
  t/1 -> Gain/1, MATLAB Function/3(t)
  MATLAB Function/3(days_mission) -> days_mission/1
  Mux/1 -> MatrixMultiply/2, B_N/1, Scope/1
  Reshape/1 -> MATLAB Function1/5(r_N), MATLAB Function/1(r_N)
  gS/1 -> MATLAB Function1/2(Mat_g)
  hS/1 -> MATLAB Function1/1(Mat_h)
  Gain/1 -> MATLAB Function1/8(days_mission)
  hsv/1 -> MATLAB Function1/4(Mat_hsv)
  r_N/1 -> Reshape/1

== system euler_equation_dave/ENVIRONMENT/MAGNETIC TORQUE/magnetic_torque ==
  note: degrees
  note: degrees
  note: M = m x B
  note: degrees
  r_N : Inport
  A_N_to_B : Inport  Port=2
  t : Inport  Port=3
  MATLAB Function : MATLAB Function  TreatAsAtomicUnit=on
  N_to_B : Product  Multiplication=Matrix(*)
  constants : Subsystem
  gaussian_coefficients : Subsystem
  m : Constant  Value=[0.01; 0.05; 0.01]
  mjd2000_block : Subsystem
  nT_to_T : Gain  Gain=1e-9
  r_N_to_lat_lon_lst : Subsystem
  theta_g : Subsystem
  to_torque : matrix_library/Cross Product
      settings: SourceProductBaseCode=SL
  magnetic_torque : Outport
  wires:
  nT_to_T/1 -> N_to_B/2  "B_N"
  gaussian_coefficients/2(h_mat) -> MATLAB Function/7(h_mat)
  mjd2000_block/1(mjd2000) -> MATLAB Function/5(mjd2000)
  gaussian_coefficients/1(g_mat) -> MATLAB Function/6(g_mat)
  constants/1(we) -> theta_g/2(we)  "we"
  constants/2(t0) -> theta_g/3(t0)  "t0"
  constants/3(theta_g0) -> theta_g/4(theta_g0)  "theta_g0"
  theta_g/1(theta_g) -> r_N_to_lat_lon_lst/2(theta_g)  "theta_g"
  r_N_to_lat_lon_lst/4(alpha) -> MATLAB Function/4(alpha)  "alpha"
  r_N_to_lat_lon_lst/1(r) -> MATLAB Function/1(r)  "r"
  m/1 -> to_torque/1  "m"
  to_torque/1 -> magnetic_torque/1  "magnetic_torque"
  N_to_B/1 -> to_torque/2  "B_B"
  MATLAB Function/1(B) -> nT_to_T/1  "B_N"
  A_N_to_B/1 -> N_to_B/1  "A_N_to_B"
  r_N_to_lat_lon_lst/3(lon) -> MATLAB Function/3(lon)  "lon"
  r_N_to_lat_lon_lst/2(lat) -> MATLAB Function/2(lat)  "lat"
  r_N/1 -> r_N_to_lat_lon_lst/1(r_N)  "r_N"
  t/1 -> theta_g/1(t)

== system euler_equation_dave/ENVIRONMENT/ORBITAL MECHANICS /cartesian position integrator ==
  Divide : Product  Inputs=*/
  Dot Product1 : DotProduct  InputSameDT=on  OutDataTypeStr=Inherit: Inherit via internal rule
  Gan : Gain  Gain=-muP
  Integrator : Integrator  InitialCondition=v0
  Integrator1 : Integrator  InitialCondition=r0
  Normalize Vector1 : vrlib/Utilities/Normalize Vector  maxzero=0
  carteasion_position_versor : Outport
  cartesian position : Outport  Port=2
  wires:
  Integrator1/1 -> cartesian position/1, Dot Product1/1, Dot Product1/2, Normalize Vector1/1  "cartesian position"
  Normalize Vector1/1 -> carteasion_position_versor/1, Divide/1  "r_versor"
  Divide/1 -> Gan/1
  Dot Product1/1 -> Divide/2  "r^2"
  Integrator/1 -> Integrator1/1
  Gan/1 -> Integrator/1  "acc"

== system euler_equation_dave/ENVIRONMENT/ORBITAL MECHANICS /cartesian position with keplerian formulas  ==
  Cos : Trigonometry  Operator=cos
  Cos1 : Trigonometry  Operator=cos
  Mux : Mux  Inputs=3
  Normalize Vector : vrlib/Utilities/Normalize Vector  maxzero=0
  Product : Product
  Product1 : Product
  Product2 : Product
  Scope : Scope
  Sin : Trigonometry
  Sin1 : Trigonometry
  eccentricity : Constant  Value=e
  inclination : Constant  Value=i_0
  to compute R : Subsystem
  to compute true anomaly : Subsystem
  R : Outport
  rN : Outport  Port=2
  r_N_versor : Outport  Port=3
  wires:
  inclination/1 -> Sin1/1, Cos1/1
  to compute true anomaly/1(theta) -> Sin/1, Cos/1, to compute R/2(theta)
  Sin/1 -> Product2/1, Product1/1
  to compute R/1(R) -> Scope/1, R/1, Product/1
  eccentricity/1 -> to compute R/1(e), to compute true anomaly/1(e)
  Cos/1 -> Mux/1
  Product/1 -> rN/1, Normalize Vector/1  "rN"
  Mux/1 -> Product/2
  Sin1/1 -> Product2/2
  Product1/1 -> Mux/2
  Cos1/1 -> Product1/2
  Product2/1 -> Mux/3
  Normalize Vector/1 -> r_N_versor/1

== system euler_equation_dave/ENVIRONMENT/To create A_L//N/To comput theta_versor ==
  h_versor : Inport
  r_N_versor : Inport  Port=2
  Cross Product : matrix_library/Cross Product
      settings: SourceProductBaseCode=SL
  Normalize Vector : vrlib/Utilities/Normalize Vector  maxzero=0
  theta_versor : Outport
  wires:
  Normalize Vector/1 -> Cross Product/2
  h_versor/1 -> Cross Product/1
  Cross Product/1 -> theta_versor/1
  r_N_versor/1 -> Normalize Vector/1

== system euler_equation_dave/KINEMATICS/KINEMATICS_EULER_ANGLES/EULER ANGLES 131 ==
  omega : Inport
  Integrator1 : Integrator  InitialCondition=Euler0131  WrapState=on
  Mux3 : Mux  Inputs=3
  PHI_DOT1 : Subsystem
  PSI DOT1 : Subsystem
  THETA DOT1 : Subsystem
  Out1 : Outport
  wires:
  Mux3/1 -> Integrator1/1
  PHI_DOT1/1(phi_dot) -> Mux3/2
  Integrator1/1 -> Out1/1, PSI DOT1/1(Euler angles), PHI_DOT1/1(euler angles), THETA DOT1/1(euler angles)
  THETA DOT1/1(theta_dot) -> Mux3/1
  omega/1 -> THETA DOT1/2(omega), PHI_DOT1/2(omega), PSI DOT1/2(omega)
  PSI DOT1/1(psi_dot) -> Mux3/3

== system euler_equation_dave/KINEMATICS/KINEMATICS_EULER_ANGLES/EULER ANGLES 312 ==
  omega : Inport
  Integrator : Integrator  InitialCondition=Euler0312  WrapState=on
  Mux2 : Mux  Inputs=3
  PHI_DOT : Subsystem
  PSI DOT : Subsystem
  THETA DOT : Subsystem
  angles : Outport
  dots : Outport  Port=2
  wires:
  omega/1 -> PSI DOT/2(omega), PHI_DOT/2(omega), THETA DOT/2(omega)
  Integrator/1 -> angles/1, PSI DOT/1(Euler angles), THETA DOT/1(euler angles), PHI_DOT/1(euler angles)
  PSI DOT/1(psi_dot) -> Mux2/3
  Mux2/1 -> dots/1, Integrator/1
  PHI_DOT/1(phi_dot) -> Mux2/1
  THETA DOT/1(theta_dot) -> Mux2/2

== system euler_equation_dave/KINEMATICS/KINEMATICS_EULER_ANGLES/If Action Subsystem ==
  phi : Inport
  theta : Inport  Port=2
  psi : Inport  Port=3
  Action Port : ActionPort  ActionPortLabel=if(u1 > - 80 & u1 < 80)
  A_312 : Subsystem
  Mux : Mux  Inputs=3
  Rotation Angles to Direction Cosine Matrix : sharedtransform/Rotation Angles to Direction Cosine Matrix  rotationOrder=ZXY  aMode=aMode
      settings: SourceProductBaseCode=AE,PW,DR,MT,UV,VE
  Scope : Scope
  Scope1 : Scope
  Sum : Sum  Inputs=-+
  A 312 : Outport
  Euler angles 312 : Outport  Port=2
  wires:
  A_312/1(A_312) -> Sum/2, A 312/1
  phi/1 -> Mux/1, A_312/1(phi)
  theta/1 -> Mux/2, A_312/2(theta)
  psi/1 -> Mux/3, A_312/3(psi)
  Mux/1 -> Rotation Angles to Direction Cosine Matrix/1, Euler angles 312/1
  Rotation Angles to Direction Cosine Matrix/1 -> Scope/1, Sum/1
  Sum/1 -> Scope1/1  "sottr"

== system euler_equation_dave/KINEMATICS/KINEMATICS_EULER_ANGLES/If Action Subsystem1 ==
  phi : Inport
  theta : Inport  Port=2
  psi : Inport  Port=3
  Action Port : ActionPort  ActionPortLabel=else
  A_131 : Subsystem
  Mux : Mux  Inputs=3
  Rotation Angles to Direction Cosine Matrix : sharedtransform/Rotation Angles to Direction Cosine Matrix  rotationOrder=XZX  aMode=aMode
      settings: SourceProductBaseCode=AE,PW,DR,MT,UV,VE
  Scope : Scope
  Sum : Sum  Inputs=+-
  A131 : Outport
  Euler angles 131 : Outport  Port=2
  wires:
  psi/1 -> Mux/3, A_131/3(psi)
  theta/1 -> Mux/2, A_131/2(theta)
  phi/1 -> Mux/1, A_131/1(phi)
  Mux/1 -> Rotation Angles to Direction Cosine Matrix/1, Euler angles 131/1
  Rotation Angles to Direction Cosine Matrix/1 -> Sum/1
  Sum/1 -> Scope/1  "sottr131"
  A_131/1(A_131) -> A131/1, Sum/2

== system euler_equation_dave/SENSORS/ATTITUDE DETERMINATION FOR GYROSCOPES/EULER ANGLES 131 ==
  omega : Inport
  Integrator1 : Integrator  InitialCondition=Euler0131  WrapState=on
  Mux3 : Mux  Inputs=3
  PHI_DOT1 : Subsystem
  PSI DOT1 : Subsystem
  THETA DOT1 : Subsystem
  Out1 : Outport
  wires:
  Mux3/1 -> Integrator1/1
  PHI_DOT1/1(phi_dot) -> Mux3/1
  Integrator1/1 -> Out1/1, PSI DOT1/1(Euler angles), THETA DOT1/1(euler angles), PHI_DOT1/1(euler angles)
  THETA DOT1/1(theta_dot) -> Mux3/2
  omega/1 -> PHI_DOT1/2(omega), THETA DOT1/2(omega), PSI DOT1/2(omega)
  PSI DOT1/1(psi_dot) -> Mux3/3

== system euler_equation_dave/SENSORS/ATTITUDE DETERMINATION FOR GYROSCOPES/EULER ANGLES 312 ==
  omega : Inport
  Integrator : Integrator  InitialCondition=Euler0312  WrapState=on
  Mux2 : Mux  Inputs=3
  PHI_DOT : Subsystem
  PSI DOT : Subsystem
  THETA DOT : Subsystem
  angles : Outport
  dots : Outport  Port=2
  wires:
  omega/1 -> PSI DOT/2(omega), PHI_DOT/2(omega), THETA DOT/2(omega)
  Integrator/1 -> angles/1, PSI DOT/1(Euler angles), THETA DOT/1(euler angles), PHI_DOT/1(euler angles)
  THETA DOT/1(theta_dot) -> Mux2/2
  PSI DOT/1(psi_dot) -> Mux2/3
  Mux2/1 -> dots/1, Integrator/1
  PHI_DOT/1(phi_dot) -> Mux2/1

== system euler_equation_dave/SENSORS/ATTITUDE DETERMINATION FOR GYROSCOPES/If Action Subsystem ==
  phi : Inport
  theta : Inport  Port=2
  psi : Inport  Port=3
  Action Port : ActionPort  ActionPortLabel=if(u1 > - 80 & u1 < 80)
  A_312 : Subsystem
  Mux : Mux  Inputs=3
  Rotation Angles to Direction Cosine Matrix : sharedtransform/Rotation Angles to Direction Cosine Matrix  rotationOrder=ZXY  aMode=aMode
      settings: SourceProductBaseCode=AE,PW,DR,MT,UV,VE
  Scope : Scope
  Scope1 : Scope
  Sum : Sum  Inputs=-+
  A 312 : Outport
  Euler angles 312 : Outport  Port=2
  wires:
  A_312/1(A_312) -> Sum/2, A 312/1
  phi/1 -> Mux/1, A_312/1(phi)
  theta/1 -> Mux/2, A_312/2(theta)
  psi/1 -> Mux/3, A_312/3(psi)
  Mux/1 -> Rotation Angles to Direction Cosine Matrix/1, Euler angles 312/1
  Rotation Angles to Direction Cosine Matrix/1 -> Scope/1, Sum/1
  Sum/1 -> Scope1/1  "sottr"

== system euler_equation_dave/SENSORS/ATTITUDE DETERMINATION FOR GYROSCOPES/If Action Subsystem1 ==
  phi : Inport
  theta : Inport  Port=2
  psi : Inport  Port=3
  Action Port : ActionPort  ActionPortLabel=else
  A_131 : Subsystem
  Mux : Mux  Inputs=3
  Rotation Angles to Direction Cosine Matrix : sharedtransform/Rotation Angles to Direction Cosine Matrix  rotationOrder=XZX  aMode=aMode
      settings: SourceProductBaseCode=AE,PW,DR,MT,UV,VE
  Scope : Scope
  Sum : Sum  Inputs=+-
  A131 : Outport
  Euler angles 131 : Outport  Port=2
  wires:
  psi/1 -> Mux/3, A_131/3(psi)
  theta/1 -> Mux/2, A_131/2(theta)
  phi/1 -> Mux/1, A_131/1(phi)
  Mux/1 -> Rotation Angles to Direction Cosine Matrix/1, Euler angles 131/1
  Rotation Angles to Direction Cosine Matrix/1 -> Sum/1
  Sum/1 -> Scope/1  "sottr131"
  A_131/1(A_131) -> A131/1, Sum/2

== system euler_equation_dave/SENSORS/GYROSCOPES/Sigma_n ==
  ARW : Constant  Value=0.0035
  Constant : Constant  Value=Ts
  Degrees to Radians1 : simulink_extras/Transformations/Degrees to Radians
  Divide : Product  Inputs=*/
  Gain1 : Gain  Gain=1/3600
  Gain2 : Gain  Gain=1/3600
  Sqrt : Sqrt  SaturateOnIntegerOverflow=on
  Out1 : Outport
  wires:
  Constant/1 -> Gain1/1
  ARW/1 -> Divide/1  "deg/sqrt(h)"
  Gain2/1 -> Out1/1
  Sqrt/1 -> Divide/2
  Gain1/1 -> Sqrt/1  "Ts in h"
  Degrees to Radians1/1 -> Gain2/1
  Divide/1 -> Degrees to Radians1/1  "sigman deg/h"

== system euler_equation_dave/ENVIRONMENT/MAGNETIC TORQUE/magnetic_torque/constants ==
  earth_rotation_speed : Constant  Value=we
  init_greenwich : Constant  Value=theta_g0
  init_time : Constant  Value=t0
  we : Outport
  t0 : Outport  Port=2
  theta_g0 : Outport  Port=3
  wires:
  earth_rotation_speed/1 -> we/1
  init_time/1 -> t0/1
  init_greenwich/1 -> theta_g0/1

== system euler_equation_dave/ENVIRONMENT/MAGNETIC TORQUE/magnetic_torque/gaussian_coefficients ==
  g : Constant  Value=g_mat
  h : Constant  Value=h_mat
  g_mat : Outport
  h_mat : Outport  Port=2
  wires:
  g/1 -> g_mat/1
  h/1 -> h_mat/1

== system euler_equation_dave/ENVIRONMENT/MAGNETIC TORQUE/magnetic_torque/mjd2000_block ==
  Clock : Clock
  Sum : Sum  Inputs=|++
  init_mjd2000 : Constant  Value=init_mjd2000
  s_to_day : Gain  Gain=1/86400
  mjd2000 : Outport
  wires:
  Sum/1 -> mjd2000/1
  s_to_day/1 -> Sum/2
  Clock/1 -> s_to_day/1
  init_mjd2000/1 -> Sum/1

== system euler_equation_dave/ENVIRONMENT/MAGNETIC TORQUE/magnetic_torque/r_N_to_lat_lon_lst ==
  r_N : Inport
  theta_g : Inport  Port=2
  Demux : Demux  Outputs=3
  latitude : Subsystem
  longitude_LST : Subsystem
      settings: PortSchema="{\"entries\":[{\"content\":{\"sides\":[{\"content\":{\"connectorIds\":[\"In1\",\"In2\",\"In3\",\"In4\"]},\"type\":\"ConnectorPlacement.EquallySpacedRectSide\",\"uuid\":\"b197dfa4-c230-4803-a0b3-2d3c44e10a73\"},{\"content\":{\"connectorIds\":[\"Out1\",\"Out2\"],\"side\":\"RIGHT\"},\"type\":\"ConnectorPlacement.EquallySpacedRectSide\",\"uuid\":\"0aaebfc3-1b92-4483-8724-e78c586dcfa0\"},{\"content\":{\"connectorIds\":[\"In5\"],\"side\":\"TOP\"},\"type\":\"ConnectorPlacement.EquallySpacedRectSide\",\"uuid\":\"07c76325-0830-48dd-a056-b0076ab4a89f\"}]},\"type\":\"ConnectorPlacement.EquallySpacedConnector\",\"uuid\":\"374bbd02-45c5-4bda-9379-dc8e2163807b\"}],\"packageUris\":[\"http://schema.mathworks.com/mf0/Connector/R2020b\"],\"version\":\"1.0\"}"
  r_norm : Subsystem  AncestorBlock=vec_norm/norm
  r : Outport
  lat : Outport  Port=2
  lon : Outport  Port=3
  alpha : Outport  Port=4
  wires:
  theta_g/1 -> longitude_LST/5(theta_g)
  longitude_LST/2(alpha) -> alpha/1  "alpha"
  longitude_LST/1(lon) -> lon/1  "lon"
  Demux/2 -> longitude_LST/3(y)  "y"
  latitude/1(lat) -> longitude_LST/4(lat), lat/1  "lat"
  Demux/3 -> latitude/2(z)  "z"
  r_norm/1(norm) -> r/1, longitude_LST/1(r), latitude/1(r)  "r"
  Demux/1 -> longitude_LST/2(x)  "x"
  r_N/1 -> Demux/1, r_norm/1(vector)  "r_N"

== system euler_equation_dave/ENVIRONMENT/MAGNETIC TORQUE/magnetic_torque/theta_g ==
  t : Inport
  we : Inport  Port=2
  t0 : Inport  Port=3
  theta_g0 : Inport  Port=4
  Product : Product
  Sum : Sum  Inputs=|++
  Sum1 : Sum  Inputs=|+-
  theta_g : Outport
  wires:
  Sum/1 -> theta_g/1  "theta_g"
  Product/1 -> Sum/1
  we/1 -> Product/1  "we"
  theta_g0/1 -> Sum/2  "theta_g0"
  t/1 -> Sum1/1  "t"
  Sum1/1 -> Product/2  "t-t0"
  t0/1 -> Sum1/2  "t0"

== system euler_equation_dave/ENVIRONMENT/ORBITAL MECHANICS /cartesian position with keplerian formulas /to compute R ==
  e : Inport
  theta : Inport  Port=2
  Constant1 : Constant
  Constant2 : Constant
  Cos1 : Trigonometry  Operator=cos
  Divide : Product  Inputs=*/
  Product : Product
  Product1 : Product
  Square : Math  Operator=square  SaturateOnIntegerOverflow=on
  Sum : Sum  Inputs=|++
  Sum1 : Sum  Inputs=+-
  semimajor axis : Constant  Value=a
  R : Outport
  wires:
  Constant2/1 -> Sum1/1
  Constant1/1 -> Sum/2
  Cos1/1 -> Product/1
  Square/1 -> Sum1/2
  Sum/1 -> Divide/2
  Product1/1 -> Divide/1
  Product/1 -> Sum/1
  semimajor axis/1 -> Product1/1
  Sum1/1 -> Product1/2
  Divide/1 -> R/1
  e/1 -> Square/1, Product/2
  theta/1 -> Cos1/1

== system euler_equation_dave/ENVIRONMENT/ORBITAL MECHANICS /cartesian position with keplerian formulas /to compute true anomaly ==
  e : Inport
  Constant1 : Constant
  Constant2 : Constant  Value=3/2
  Cos : Trigonometry  Operator=cos
  Divide : Product  Inputs=*/
  Integrator : Integrator  InitialCondition=true_anomaly0
  Math Function : Math  Operator=pow  SaturateOnIntegerOverflow=on
  Product : Product
  Product1 : Product
  Square : Math  Operator=square  SaturateOnIntegerOverflow=on
  Square1 : Math  Operator=square  SaturateOnIntegerOverflow=on
  Sum : Sum  Inputs=|++
  Sum1 : Sum  Inputs=+-
  angular velocity of orbit? : Constant  Value=n
  theta : Outport
  wires:
  Sum/1 -> Square/1
  Constant1/1 -> Sum/2, Sum1/1
  Divide/1 -> Integrator/1  "theta_dot"
  Product/1 -> Sum/1
  Cos/1 -> Product/2
  angular velocity of orbit?/1 -> Product1/1
  Product1/1 -> Divide/1
  Square1/1 -> Sum1/2
  Square/1 -> Product1/2
  Sum1/1 -> Math Function/1
  e/1 -> Square1/1, Product/1
  Math Function/1 -> Divide/2
  Integrator/1 -> theta/1, Cos/1  "theta"
  Constant2/1 -> Math Function/2

== system euler_equation_dave/KINEMATICS/KINEMATICS_EULER_ANGLES/EULER ANGLES 131/PHI_DOT1 ==
  euler angles : Inport
  omega : Inport  Port=2
  Cos : Trigonometry  Operator=cos
  Cos1 : Trigonometry
  Demux : Demux  Outputs=3
  Demux1 : Demux  Outputs=3
  Divide : Product  Inputs=*/
  Product : Product
  Product1 : Product
  Sin : Trigonometry
  Sum : Sum  Inputs=-+
  Terminator : Terminator
  Terminator1 : Terminator
  phi_dot : Outport
  wires:
  omega/1 -> Demux/1
  euler angles/1 -> Demux1/1
  Demux1/2 -> Cos1/1
  Demux1/1 -> Terminator1/1
  Demux1/3 -> Cos/1, Sin/1
  Product/1 -> Sum/1
  Product1/1 -> Sum/2
  Sum/1 -> Divide/1
  Divide/1 -> phi_dot/1
  Demux/1 -> Terminator/1
  Cos1/1 -> Divide/2  "sin_theta!"
  Demux/3 -> Product1/2
  Sin/1 -> Product1/1
  Demux/2 -> Product/2  "w2"
  Cos/1 -> Product/1

== system euler_equation_dave/KINEMATICS/KINEMATICS_EULER_ANGLES/EULER ANGLES 131/PSI DOT1 ==
  Euler angles : Inport
  omega : Inport  Port=2
  Cos : Trigonometry  Operator=cos
  Cos1 : Trigonometry  Operator=cos
  Demux : Demux  Outputs=3
  Demux1 : Demux  Outputs=3
  Divide : Product  Inputs=*/
  Product : Product
  Product1 : Product
  Product2 : Product
  Sin : Trigonometry
  Sin1 : Trigonometry
  Sum : Sum  Inputs=+-
  Sum1 : Sum
  Terminator1 : Terminator
  psi_dot : Outport
  wires:
  Demux1/3 -> Cos/1, Sin/1
  Demux1/2 -> Sin1/1, Cos1/1
  Product/1 -> Sum/1
  Demux1/1 -> Terminator1/1
  Product1/1 -> Sum/2
  Euler angles/1 -> Demux1/1
  omega/1 -> Demux/1
  Divide/1 -> Sum1/1
  Sum1/1 -> psi_dot/1
  Sum/1 -> Product2/2  "w2*cos_psi-w3*sin_psi"
  Product2/1 -> Divide/1
  Demux/1 -> Sum1/2  "w1"
  Sin1/1 -> Divide/2  "sintheta!"
  Cos1/1 -> Product2/1  "cos_theta!"
  Demux/2 -> Product/1
  Cos/1 -> Product/2
  Demux/3 -> Product1/1
  Sin/1 -> Product1/2

== system euler_equation_dave/KINEMATICS/KINEMATICS_EULER_ANGLES/EULER ANGLES 131/THETA DOT1 ==
  euler angles : Inport
  omega : Inport  Port=2
  Cos : Trigonometry  Operator=cos
  Demux : Demux  Outputs=3
  Demux1 : Demux  Outputs=3
  Product : Product
  Product1 : Product
  Sin : Trigonometry
  Sum : Sum
  Terminator : Terminator
  Terminator1 : Terminator
  Terminator2 : Terminator
  theta_dot : Outport
  wires:
  Cos/1 -> Product/1
  Demux1/3 -> Sin/1, Cos/1
  Sin/1 -> Product1/2
  Product/1 -> Sum/1  "w3*cos_psi"
  Demux1/1 -> Terminator1/1
  omega/1 -> Demux/1
  Sum/1 -> theta_dot/1
  euler angles/1 -> Demux1/1
  Product1/1 -> Sum/2  "w2*sin_psi"
  Demux1/2 -> Terminator2/1
  Demux/1 -> Terminator/1
  Demux/3 -> Product/2
  Demux/2 -> Product1/1  "w2"

== system euler_equation_dave/KINEMATICS/KINEMATICS_EULER_ANGLES/EULER ANGLES 312/PHI_DOT ==
  euler angles : Inport
  omega : Inport  Port=2
  Cos : Trigonometry  Operator=cos
  Cos1 : Trigonometry  Operator=cos
  Demux : Demux  Outputs=3
  Demux1 : Demux  Outputs=3
  Divide : Product  Inputs=*/
  Product : Product
  Product1 : Product
  Sin : Trigonometry
  Sum : Sum  Inputs=+-
  Terminator : Terminator
  Terminator1 : Terminator
  phi_dot : Outport
  wires:
  omega/1 -> Demux/1
  Demux/2 -> Terminator/1  "w2"
  Demux/1 -> Product1/1
  euler angles/1 -> Demux1/1
  Demux1/2 -> Cos1/1
  Demux1/1 -> Terminator1/1
  Demux1/3 -> Cos/1, Sin/1
  Sin/1 -> Product1/2
  Cos/1 -> Product/1
  Demux/3 -> Product/2
  Product/1 -> Sum/1
  Cos1/1 -> Divide/2  "cos_theta!"
  Product1/1 -> Sum/2
  Sum/1 -> Divide/1
  Divide/1 -> phi_dot/1

== system euler_equation_dave/KINEMATICS/KINEMATICS_EULER_ANGLES/EULER ANGLES 312/PSI DOT ==
  Euler angles : Inport
  omega : Inport  Port=2
  Cos : Trigonometry  Operator=cos
  Cos1 : Trigonometry  Operator=cos
  Demux : Demux  Outputs=3
  Demux1 : Demux  Outputs=3
  Divide : Product  Inputs=*/
  Product : Product
  Product1 : Product
  Product2 : Product
  Sin : Trigonometry
  Sin1 : Trigonometry
  Sum : Sum  Inputs=+-
  Sum1 : Sum  Inputs=-+
  Terminator1 : Terminator
  psi_dot : Outport
  wires:
  Demux1/3 -> Cos/1, Sin/1
  Demux1/2 -> Sin1/1, Cos1/1
  Product/1 -> Sum/1
  Demux1/1 -> Terminator1/1
  Cos1/1 -> Divide/2  "cos_theta!"
  Product1/1 -> Sum/2
  Euler angles/1 -> Demux1/1
  omega/1 -> Demux/1
  Demux/2 -> Sum1/2  "w2"
  Divide/1 -> Sum1/1
  Sum1/1 -> psi_dot/1
  Demux/3 -> Product/2
  Cos/1 -> Product/1
  Demux/1 -> Product1/1
  Sin/1 -> Product1/2
  Sin1/1 -> Product2/1
  Sum/1 -> Product2/2  "w3*cos_psi-w1*sin_psi"
  Product2/1 -> Divide/1

== system euler_equation_dave/KINEMATICS/KINEMATICS_EULER_ANGLES/EULER ANGLES 312/THETA DOT ==
  euler angles : Inport
  omega : Inport  Port=2
  Cos : Trigonometry  Operator=cos
  Demux : Demux  Outputs=3
  Demux1 : Demux  Outputs=3
  Product : Product
  Product1 : Product
  Sin : Trigonometry
  Sum : Sum
  Terminator : Terminator
  Terminator1 : Terminator
  Terminator2 : Terminator
  theta_dot : Outport
  wires:
  Cos/1 -> Product/1
  Demux/2 -> Terminator/1  "w2"
  Demux1/3 -> Sin/1, Cos/1
  Sin/1 -> Product1/2
  Product/1 -> Sum/1  "w1*cos_psi"
  Demux1/1 -> Terminator1/1
  omega/1 -> Demux/1
  Sum/1 -> theta_dot/1
  euler angles/1 -> Demux1/1
  Product1/1 -> Sum/2  "w3*sin_psi"
  Demux1/2 -> Terminator2/1
  Demux/1 -> Product/2
  Demux/3 -> Product1/1
